simulink model "dz3_6dof_ned_compare"  (R2026a)
settings: Solver=ode4  StopTime=4  FixedStep=0.001
InitFcn:
  | dz3ProjectRoot = fileparts(fileparts(get_param(bdroot,'FileName'))); addpath(fullfile(dz3ProjectRoot,'scripts'));                         dz3_init_default_inputs(bdroot);
libraries: aerolibprivatev1p5 x1
settings Model: Creator=ievge  LastModifiedBy=ievge

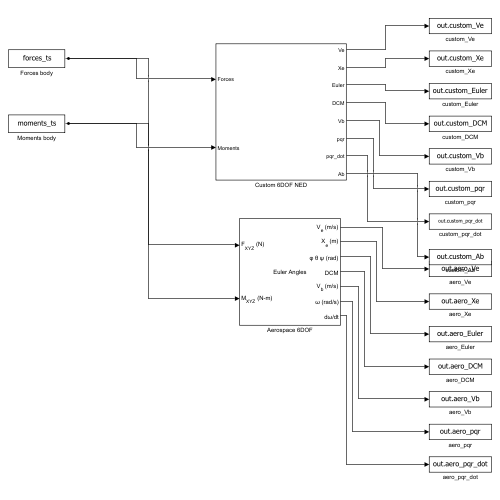
[thumbnail: Simulink's stored preview of the top-level diagram]
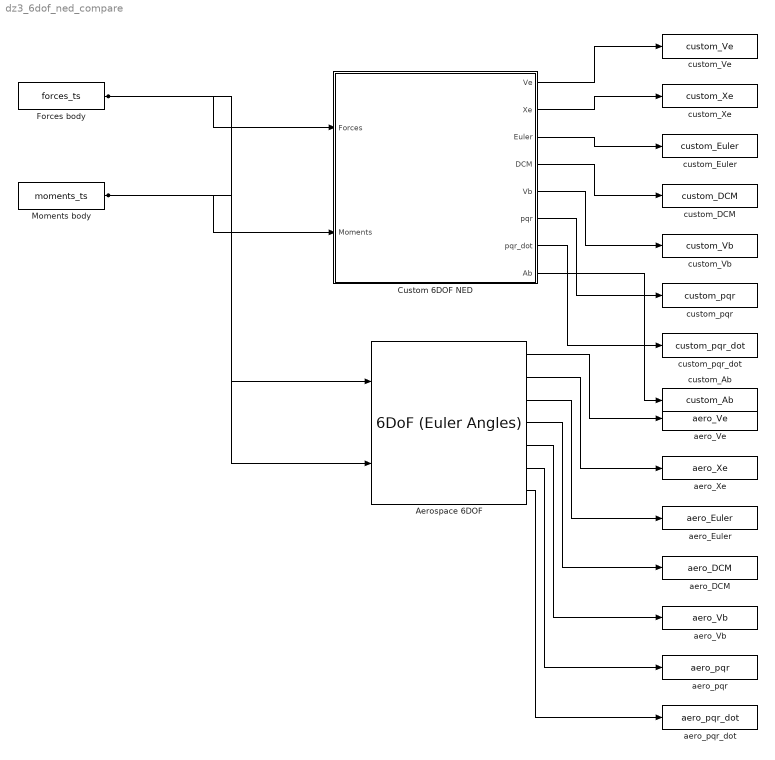
== system dz3_6dof_ned_compare ==
  Aerospace 6DOF : aerolibprivatev1p5/6DoF (Euler Angles)  xme_0=[0;0;-10]  Vm_0=[0;0;0]  eul_0=[0;0;0]  pm_0=[0;0;0]  Mass=1.3211359852721711  Inertia=diag([0.0093 0.0092 0.0151])
  Custom 6DOF NED : Subsystem
  Forces body : FromWorkspace  VariableName=forces_ts
  Moments body : FromWorkspace  VariableName=moments_ts
  aero_DCM : ToWorkspace  VariableName=aero_DCM  SaveFormat=Timeseries  SampleTime=-1
  aero_Euler : ToWorkspace  VariableName=aero_Euler  SaveFormat=Timeseries  SampleTime=-1
  aero_Vb : ToWorkspace  VariableName=aero_Vb  SaveFormat=Timeseries  SampleTime=-1
  aero_Ve : ToWorkspace  VariableName=aero_Ve  SaveFormat=Timeseries  SampleTime=-1
  aero_Xe : ToWorkspace  VariableName=aero_Xe  SaveFormat=Timeseries  SampleTime=-1
  aero_pqr : ToWorkspace  VariableName=aero_pqr  SaveFormat=Timeseries  SampleTime=-1
  aero_pqr_dot : ToWorkspace  VariableName=aero_pqr_dot  SaveFormat=Timeseries  SampleTime=-1
  custom_Ab : ToWorkspace  VariableName=custom_Ab  SaveFormat=Timeseries  SampleTime=-1
  custom_DCM : ToWorkspace  VariableName=custom_DCM  SaveFormat=Timeseries  SampleTime=-1
  custom_Euler : ToWorkspace  VariableName=custom_Euler  SaveFormat=Timeseries  SampleTime=-1
  custom_Vb : ToWorkspace  VariableName=custom_Vb  SaveFormat=Timeseries  SampleTime=-1
  custom_Ve : ToWorkspace  VariableName=custom_Ve  SaveFormat=Timeseries  SampleTime=-1
  custom_Xe : ToWorkspace  VariableName=custom_Xe  SaveFormat=Timeseries  SampleTime=-1
  custom_pqr : ToWorkspace  VariableName=custom_pqr  SaveFormat=Timeseries  SampleTime=-1
  custom_pqr_dot : ToWorkspace  VariableName=custom_pqr_dot  SaveFormat=Timeseries  SampleTime=-1
  wires:
  Forces body/1 -> Custom 6DOF NED/1(Forces), Aerospace 6DOF/1
  Moments body/1 -> Custom 6DOF NED/2(Moments), Aerospace 6DOF/2
  Custom 6DOF NED/1(Ve) -> custom_Ve/1
  Aerospace 6DOF/1 -> aero_Ve/1
  Custom 6DOF NED/2(Xe) -> custom_Xe/1
  Aerospace 6DOF/2 -> aero_Xe/1
  Custom 6DOF NED/3(Euler) -> custom_Euler/1
  Aerospace 6DOF/3 -> aero_Euler/1
  Custom 6DOF NED/4(DCM) -> custom_DCM/1
  Aerospace 6DOF/4 -> aero_DCM/1
  Custom 6DOF NED/5(Vb) -> custom_Vb/1
  Aerospace 6DOF/5 -> aero_Vb/1
  Custom 6DOF NED/6(pqr) -> custom_pqr/1
  Aerospace 6DOF/6 -> aero_pqr/1
  Custom 6DOF NED/7(pqr_dot) -> custom_pqr_dot/1
  Aerospace 6DOF/7 -> aero_pqr_dot/1
  Custom 6DOF NED/8(Ab) -> custom_Ab/1

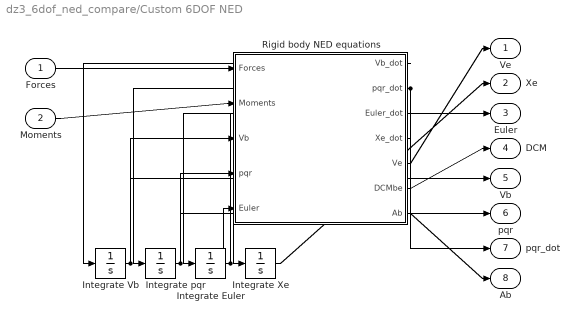
== system dz3_6dof_ned_compare/Custom 6DOF NED ==
  Forces : Inport
  Moments : Inport  Port=2
  Integrate Euler : Integrator  InitialCondition=[0;0;0]
  Integrate Vb : Integrator  InitialCondition=[0;0;0]
  Integrate Xe : Integrator  InitialCondition=[0;0;-10]
  Integrate pqr : Integrator  InitialCondition=[0;0;0]
  Rigid body NED equations : MATLAB Function  TreatAsAtomicUnit=on
  Ve : Outport
  Xe : Outport  Port=2
  Euler : Outport  Port=3
  DCM : Outport  Port=4
  Vb : Outport  Port=5
  pqr : Outport  Port=6
  pqr_dot : Outport  Port=7
  Ab : Outport  Port=8
  wires:
  ? -> ?
  Forces/1 -> Rigid body NED equations/1(Forces)
  Moments/1 -> Rigid body NED equations/2(Moments)
  Integrate Vb/1 -> Rigid body NED equations/3(Vb), Vb/1
  Integrate pqr/1 -> Rigid body NED equations/4(pqr), pqr/1
  Integrate Euler/1 -> Rigid body NED equations/5(Euler), Euler/1
  Rigid body NED equations/1(Vb_dot) -> Integrate Vb/1
  Rigid body NED equations/2(pqr_dot) -> Integrate pqr/1, pqr_dot/1
  Rigid body NED equations/3(Euler_dot) -> Integrate Euler/1
  Rigid body NED equations/4(Xe_dot) -> Integrate Xe/1
  Rigid body NED equations/5(Ve) -> Ve/1
  Integrate Xe/1 -> Xe/1
  Rigid body NED equations/6(DCMbe) -> DCM/1
  Rigid body NED equations/7(Ab) -> Ab/1

== matlab function dz3_6dof_ned_compare/Custom 6DOF NED/Rigid body NED equations ==
  data: Forces input; Vb_dot output; Moments input; Vb input; pqr input; Euler input; pqr_dot output; Euler_dot output; Xe_dot output; Ve output; DCMbe output; Ab output
function [Vb_dot,pqr_dot,Euler_dot,Xe_dot,Ve,DCMbe,Ab] = fcn(Forces,Moments,Vb,pqr,Euler)
% 6DOF rigid-body equations, body axes + NED navigation frame.
Forces = Forces(:); Moments = Moments(:); Vb = Vb(:); pqr = pqr(:); Euler = Euler(:);
mass = 1.3211359852721711;
I = diag([0.0093 0.0092 0.0151]);
phi = Euler(1); theta = Euler(2); psi = Euler(3);
cphi = cos(phi); sphi = sin(phi); ctheta = cos(theta); stheta = sin(theta);
cpsi = cos(psi); spsi = sin(psi);
DCMbe = [ctheta*cpsi, ctheta*spsi, -stheta; sphi*stheta*cpsi-cphi*spsi, sphi*stheta*spsi+cphi*cpsi, sphi*ctheta; cphi*stheta*cpsi+sphi*spsi, cphi*stheta*spsi-sphi*cpsi, cphi*ctheta];
Ab = Forces/mass - cross(pqr,Vb);
pqr_dot = I \ (Moments - cross(pqr,I*pqr));
Euler_dot = [1, sphi*tan(theta), cphi*tan(theta); 0, cphi, -sphi; 0, sphi/ctheta, cphi/ctheta]*pqr;
Ve = DCMbe.'*Vb;
Xe_dot = Ve;
Vb_dot = Ab;
end
